simulink model "PMSMSystem"  (R2022b)
settings: Solver=FixedStepAuto  StartTime=0.0  StopTime=10.0  FixedStep=1e-3  RelTol=1e-3
model workspace (MAT data in the model file):
  Lm = 0.02
  Lr = 0.005
  Ls = 0.01
  P = 2
  R = 1
  Sig = Simulink.Signal
  Sig.DataType = 'auto'
  Sig.Dimensions = -1
  Sig.DimensionsMode = 'auto'
  Sig.Complexity = 'auto'
  Sig.SampleTime = -1
  Sig.SamplingMode = 'auto'
  gama = 0.1
settings Model: Creator=MAAM  LastModifiedBy=MAAM

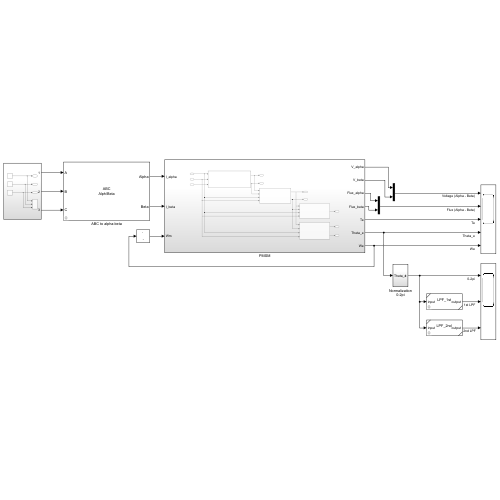
[thumbnail: Simulink's stored preview of the top-level diagram]
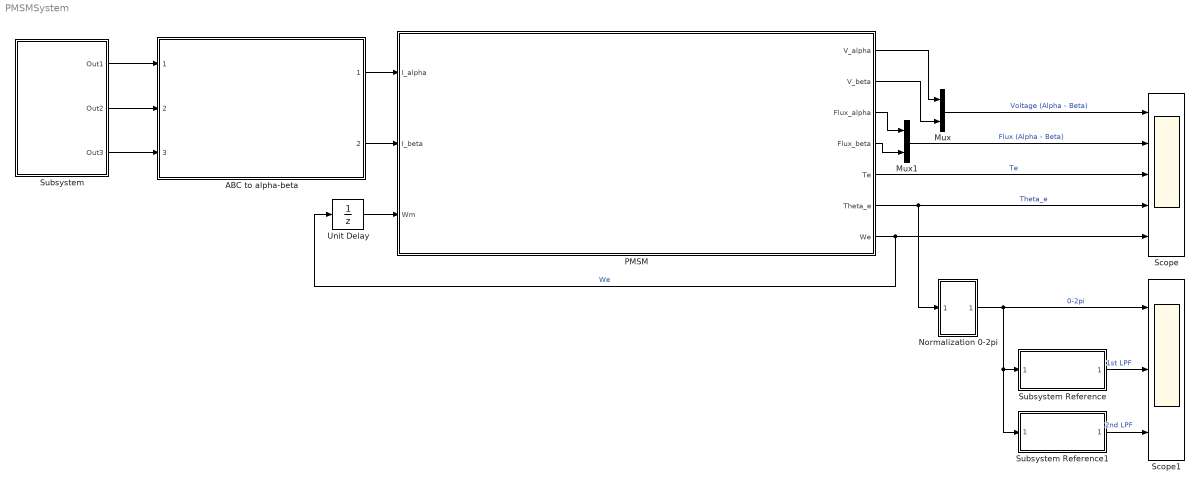
== system PMSMSystem ==
  ABC to alpha-beta : Subsystem  ReferencedSubsystem=ABC_to_alpha_beta
  Mux : Mux  Inputs=2
  Mux1 : Mux  Inputs=2
  Normalization 0-2pi : Subsystem
  PMSM : Subsystem
  Scope : Scope  NumInputPorts=5
  Scope1 : Scope  NumInputPorts=3
  Subsystem : Subsystem
  Subsystem Reference : Subsystem  ReferencedSubsystem=LPF_1st  fc=300/(2*pi)  wc=300
  Subsystem Reference1 : Subsystem  ReferencedSubsystem=LPF_2nd  fc=300/(2*pi)  w0=300  e=1/sqrt(2)
  Unit Delay : UnitDelay  SampleTime=-1  HasFrameUpgradeWarning=on
  wires:
  Subsystem/1(Out1) -> ABC to alpha-beta/1
  Subsystem/2(Out2) -> ABC to alpha-beta/2
  Subsystem/3(Out3) -> ABC to alpha-beta/3
  PMSM/7(We) -> Unit Delay/1, Scope/5  "We"
  Unit Delay/1 -> PMSM/3(Wm)
  ABC to alpha-beta/2 -> PMSM/2(I_beta)
  ABC to alpha-beta/1 -> PMSM/1(I_alpha)
  PMSM/1(V_alpha) -> Mux/1
  PMSM/2(V_beta) -> Mux/2
  PMSM/3(Flux_alpha) -> Mux1/1
  PMSM/4(Flux_beta) -> Mux1/2
  Mux/1 -> Scope/1  "Voltage (Alpha - Beta)"
  Mux1/1 -> Scope/2  "Flux (Alpha - Beta)"
  PMSM/5(Te) -> Scope/3  "Te"
  PMSM/6(Theta_e) -> Scope/4, Normalization 0-2pi/1(Theta_e)  "Theta_e"
  Normalization 0-2pi/1(Out1) -> Subsystem Reference1/1, Subsystem Reference/1, Scope1/1  "0-2pi"
  Subsystem Reference/1 -> Scope1/2  "1st LPF"
  Subsystem Reference1/1 -> Scope1/3  "2nd LPF"

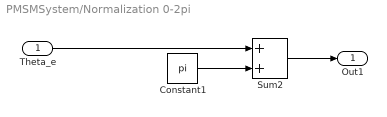
== system PMSMSystem/Normalization 0-2pi ==
  Theta_e : Inport
  Constant1 : Constant  Value=pi
  Sum2 : Sum
  Out1 : Outport
  wires:
  Constant1/1 -> Sum2/2
  Sum2/1 -> Out1/1
  Theta_e/1 -> Sum2/1

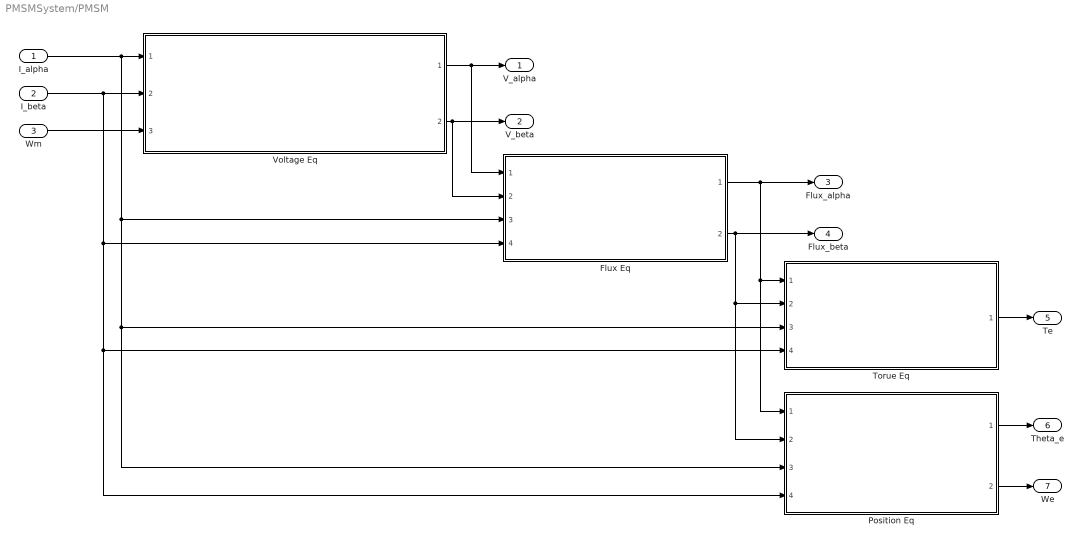
== system PMSMSystem/PMSM ==
  I_alpha : Inport
  I_beta : Inport  Port=2
  Wm : Inport  Port=3
  Flux Eq : Subsystem  ReferencedSubsystem=Flux_Eq  R=R  Ls=Ls
  Position Eq : Subsystem  ReferencedSubsystem=Position_Eq
  Torue Eq : Subsystem  ReferencedSubsystem=Torue_Eq  P=P
  Voltage Eq : Subsystem  ReferencedSubsystem=Voltage_Eq  R=R  Ls=Ls  Lr=Lr
  V_alpha : Outport
  V_beta : Outport  Port=2
  Flux_alpha : Outport  Port=3
  Flux_beta : Outport  Port=4
  Te : Outport  Port=5
  Theta_e : Outport  Port=6
  We : Outport  Port=7
  wires:
  I_alpha/1 -> Position Eq/3, Torue Eq/3, Flux Eq/3, Voltage Eq/1
  Wm/1 -> Voltage Eq/3
  Voltage Eq/1 -> V_alpha/1, Flux Eq/1
  Voltage Eq/2 -> V_beta/1, Flux Eq/2
  I_beta/1 -> Position Eq/4, Torue Eq/4, Flux Eq/4, Voltage Eq/2
  Flux Eq/1 -> Position Eq/1, Torue Eq/1, Flux_alpha/1
  Flux Eq/2 -> Flux_beta/1, Torue Eq/2, Position Eq/2
  Torue Eq/1 -> Te/1
  Position Eq/1 -> Theta_e/1
  Position Eq/2 -> We/1

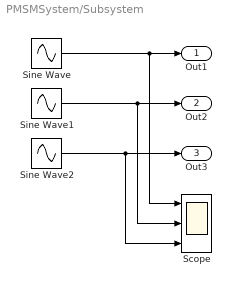
== system PMSMSystem/Subsystem ==
  Scope : Scope  NumInputPorts=3
  Sine Wave : Sin  Amplitude=2  Frequency=300  Phase=0*(pi/180)  SampleTime=0
  Sine Wave1 : Sin  Amplitude=2  Frequency=300  Phase=-120*(pi/180)  SampleTime=0
  Sine Wave2 : Sin  Amplitude=2  Frequency=300  Phase=120*(pi/180)  SampleTime=0
  Out1 : Outport
  Out2 : Outport  Port=2
  Out3 : Outport  Port=3
  wires:
  Sine Wave/1 -> Out1/1, Scope/1
  Sine Wave1/1 -> Out2/1, Scope/2
  Sine Wave2/1 -> Out3/1, Scope/3
